simulink model "ConfiguredVirtualVehicleModel"  (R2023b)
settings: configuration reference "VehicleVariable" (kept outside this file)
StartFcn:
  | %tic
StopFcn:
  | %toc
model workspace (MAT data in the model file):
  ExtDrvCmdsSwitch : Simulink.Parameter (value not decoded)
  ExtDrvRefSwitch : Simulink.Parameter (value not decoded)
  ExtEnvSwitch : Simulink.Parameter (value not decoded)
  ExtGndSwitch : Simulink.Parameter (value not decoded)
values from neighbouring files (symbols this model uses):
  L = 2.79    [EVFmincon_custom.m]
symbols that are objects in the model workspace (value not decoded): ExtDrvCmdsSwitch, ExtDrvRefSwitch, ExtEnvSwitch, ExtGndSwitch
undefined symbols (not defined in the file or in its folder): AccelCmd, AmbTemp, BaroPress, CtrlTcuInitGear, CtrlVcuCltch1InitCmd, CurvGradRef, CurvRef, DCM, DecelCmd, Disabled, DriverAeroRes, DriverDrivelineRes, DriverInitialGear, DriverPreviewDist, DriverRollRes, DriverShiftTime, DriverTimeConst, DriverTractiveForce, EnvAbsPrs, EnvAirTemp, EnvGrvty, EnvNomFrictionScaling, EnvNominalGrade, EnvWindVelX, EnvWindVelY, EnvWindVelZ, FTP75, Gnd, Grade, HazzardCmd, HighBeamCmd, lambda_mux, LeftSignalCmd, LngRef, LowBeamCmd, LtrRef, PhiRef, PlntVehDstCGFrntAxl, PlntVehDstCGRearAxl, PlntVehInitLatPos, PlntVehInitLongPos, PlntVehInitPitchAng, PlntVehInitRollAng, PlntVehInitVertPos, PlntVehInitYawAng, PlntVehMass, PlntVehTrckWdth, PlntVehYawMomentInertia, PlntWhlLdRadius, RightSignalCmd, ScnCRMaxLatAccel, ScnCRRadius, ScnDLCGateLongPos, ScnDLCLatRef, ScnDLCLatRefOffset, ScnDLCLongRefBpt, ScnDLCLongRefStartPos, ScnDLCVehicleWidth, ScnFHCounterDwellTime, ScnFHInitialDwellTime ... (+22)
libraries: simulink x27, autolibutils x8, vehdynlibscenariocommon x7, vehdynlibviscommon x3, vehdynlibdriver x2, sim3dgroundtruthsensorlib x2, autolibshared x2, vrlib x1, autolibsharedcommon x1, sharedtransform x1, sim3dlib x1, sim3dautolib x1
(part 2 of 6)

== system ConfiguredVirtualVehicleModel/Controllers/Thermal Management ==
  CoolTemp : Inport
  CellTemps : Inport  Port=2
  No Control : Subsystem  VariantControl=No Control
  Thermal Control : ModelReference  ModelNameDialog=ThermalControl.slx  SimulationMode=Normal  VariantControl=Thermal Control  ModelReferenceVersion=1.43
  ValveCmd : Outport
  PumpCmd : Outport  Port=2

== system ConfiguredVirtualVehicleModel/Controllers/Thermal Output ==
  ValveCmd : Inport
  PumpCmd : Inport  Port=2
  Bus Creator : BusCreator  Inputs=2
  Thermal : Outport
  wires:
  PumpCmd/1 -> Bus Creator/2  "PumpCmd"
  ValveCmd/1 -> Bus Creator/1  "ValveCmd"
  Bus Creator/1 -> Thermal/1

== system ConfiguredVirtualVehicleModel/Controllers/Transmission Control Unit (TCU) ==
  Accel : Inport
  BrkCmd : Inport  Port=2
  GearReq : Inport  Port=3
  EngSpd : Inport  Port=4
  Omega : Inport  Port=5  Unit=rad/s
  VehSpdFdbk : Inport  Port=6
  ABSFlag : Inport  Port=7
  UpReq : Inport  Port=8
  DownReq : Inport  Port=9  Unit=rad/s
  DriverPassThrough : ModelReference  ModelNameDialog=DriverPassThrough  SimulationMode=Normal  VariantControl=DriverPassThrough  ModelReferenceVersion=7.0
  " Gear" : Outport  VectorParamsAs1DForOutWhenUnconnected=off

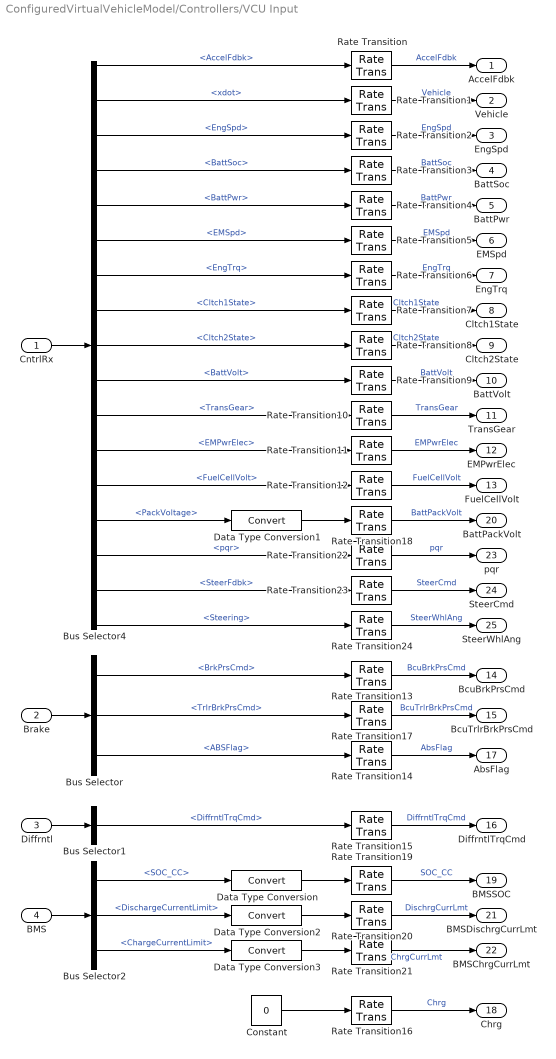
== system ConfiguredVirtualVehicleModel/Controllers/VCU Input ==
  CntrlRx : Inport
  Brake : Inport  Port=2
  Diffrntl : Inport  Port=3
  BMS : Inport  Port=4
  Bus Selector : BusSelector  OutputSignals=BrkPrsCmd,TrlrBrkPrsCmd,ABSFlag
  Bus Selector1 : BusSelector  OutputSignals=DiffrntlTrqCmd
  Bus Selector2 : BusSelector  OutputSignals=BMSInfo.SOC.SOC_CC,BMSCmd.CurrentLimitsBus.DischargeCurrentLimit,BMSCmd.CurrentLimitsBus.ChargeCurrentLimit
  Bus Selector4 : BusSelector  OutputSignals=Driver.AccelFdbk,Vehicle.xdot,Trans.EngSpd,Battery.BattSoc,Battery.BattPwr,Trans.EMSpd,Engine.EngTrq,Trans.Cltch1State,Trans.Cltch2State,Battery.BattVolt,Trans.TransGear,EM.EMPwrElec,FuelCell.FuelCellVolt,Battery.BMSSensors.PackVoltage,IMU.pqr,Driver.SteerFdbk,Steering
  Constant : Constant  Value=0  SampleTime=-1
  Data Type Conversion{,1..3} (4 alike) : DataTypeConversion  SaturateOnIntegerOverflow=off  RndMeth=Floor
  Rate Transition{,1..24} (25 alike) : RateTransition  Deterministic=off
  AccelFdbk : Outport
  Vehicle : Outport  Port=2
  EngSpd : Outport  Port=3
  BattSoc : Outport  Port=4
  BattPwr : Outport  Port=5
  EMSpd : Outport  Port=6
  EngTrq : Outport  Port=7
  Cltch1State : Outport  Port=8
  Cltch2State : Outport  Port=9
  BattVolt : Outport  Port=10
  TransGear : Outport  Port=11
  EMPwrElec : Outport  Port=12
  FuelCellVolt : Outport  Port=13
  BcuBrkPrsCmd : Outport  Port=14
  BcuTrlrBrkPrsCmd : Outport  Port=15
  DiffrntlTrqCmd : Outport  Port=16
  AbsFlag : Outport  Port=17
  Chrg : Outport  Port=18
  BMSSOC : Outport  Port=19
  BattPackVolt : Outport  Port=20
  BMSDischrgCurrLmt : Outport  Port=21
  BMSChrgCurrLmt : Outport  Port=22
  pqr : Outport  Port=23
  SteerCmd : Outport  Port=24
  SteerWhlAng : Outport  Port=25
  wires:
  Bus Selector4/5 -> Rate Transition4/1  "<BattPwr>"
  Bus Selector4/1 -> Rate Transition/1  "<AccelFdbk>"
  Bus Selector4/7 -> Rate Transition6/1  "<EngTrq>"
  Bus Selector4/4 -> Rate Transition3/1  "<BattSoc>"
  Bus Selector4/6 -> Rate Transition5/1  "<EMSpd>"
  CntrlRx/1 -> Bus Selector4/1
  Bus Selector4/11 -> Rate Transition10/1  "<TransGear>"
  Bus Selector4/9 -> Rate Transition8/1  "<Cltch2State>"
  Bus Selector4/13 -> Rate Transition12/1  "<FuelCellVolt>"
  Bus Selector4/2 -> Rate Transition1/1  "<xdot>"
  Bus Selector4/8 -> Rate Transition7/1  "<Cltch1State>"
  Bus Selector4/10 -> Rate Transition9/1  "<BattVolt>"
  Bus Selector4/3 -> Rate Transition2/1  "<EngSpd>"
  Bus Selector4/12 -> Rate Transition11/1  "<EMPwrElec>"
  Bus Selector/1 -> Rate Transition13/1  "<BrkPrsCmd>"
  Constant/1 -> Rate Transition16/1
  Brake/1 -> Bus Selector/1
  Bus Selector/3 -> Rate Transition14/1  "<ABSFlag>"
  Diffrntl/1 -> Bus Selector1/1
  Bus Selector1/1 -> Rate Transition15/1  "<DiffrntlTrqCmd>"
  Rate Transition/1 -> AccelFdbk/1  "AccelFdbk"
  Rate Transition1/1 -> Vehicle/1  "Vehicle"
  Rate Transition2/1 -> EngSpd/1  "EngSpd"
  Rate Transition3/1 -> BattSoc/1  "BattSoc"
  Rate Transition4/1 -> BattPwr/1  "BattPwr"
  Rate Transition5/1 -> EMSpd/1  "EMSpd"
  Rate Transition6/1 -> EngTrq/1  "EngTrq"
  Rate Transition7/1 -> Cltch1State/1  "Cltch1State"
  Rate Transition8/1 -> Cltch2State/1  "Cltch2State"
  Rate Transition9/1 -> BattVolt/1  "BattVolt"
  Rate Transition10/1 -> TransGear/1  "TransGear"
  Rate Transition11/1 -> EMPwrElec/1  "EMPwrElec"
  Rate Transition12/1 -> FuelCellVolt/1  "FuelCellVolt"
  Rate Transition13/1 -> BcuBrkPrsCmd/1  "BcuBrkPrsCmd"
  Rate Transition14/1 -> AbsFlag/1  "AbsFlag"
  Rate Transition15/1 -> DiffrntlTrqCmd/1  "DiffrntlTrqCmd"
  Rate Transition16/1 -> Chrg/1  "Chrg"
  Rate Transition20/1 -> BMSDischrgCurrLmt/1  "DischrgCurrLmt"
  Rate Transition19/1 -> BMSSOC/1  "SOC_CC"
  Rate Transition21/1 -> BMSChrgCurrLmt/1  "ChrgCurrLmt"
  Data Type Conversion3/1 -> Rate Transition21/1
  Data Type Conversion2/1 -> Rate Transition20/1
  Bus Selector2/1 -> Data Type Conversion/1  "<SOC_CC>"
  Data Type Conversion/1 -> Rate Transition19/1
  Bus Selector2/3 -> Data Type Conversion3/1  "<ChargeCurrentLimit>"
  Bus Selector2/2 -> Data Type Conversion2/1  "<DischargeCurrentLimit>"
  BMS/1 -> Bus Selector2/1
  Data Type Conversion1/1 -> Rate Transition18/1
  Rate Transition18/1 -> BattPackVolt/1  "BattPackVolt"
  Bus Selector4/14 -> Data Type Conversion1/1  "<PackVoltage>"
  Bus Selector/2 -> Rate Transition17/1  "<TrlrBrkPrsCmd>"
  Rate Transition17/1 -> BcuTrlrBrkPrsCmd/1  "BcuTrlrBrkPrsCmd"
  Rate Transition22/1 -> pqr/1  "pqr"
  Rate Transition23/1 -> SteerCmd/1  "SteerCmd"
  Rate Transition24/1 -> SteerWhlAng/1  "SteerWhlAng"
  Bus Selector4/15 -> Rate Transition22/1  "<pqr>"
  Bus Selector4/16 -> Rate Transition23/1  "<SteerFdbk>"
  Bus Selector4/17 -> Rate Transition24/1  "<Steering>"

== system ConfiguredVirtualVehicleModel/Controllers/VCU Output ==
  EngTrqCmd : Inport
  EMTrqCmd : Inport  Port=2
  VcuBrkPrsCmd : Inport  Port=3
  VcuTrlrBrkPrsCmd : Inport  Port=4
  Cltch1Cmd : Inport  Port=5
  Neutral : Inport  Port=6
  FuelCellCurrCmd : Inport  Port=7
  FuelCellTempCmd : Inport  Port=8
  Bus Creator5 : BusCreator  Inputs=8
  Vcu : Outport
  wires:
  Cltch1Cmd/1 -> Bus Creator5/5  "Cltch1Cmd"
  EngTrqCmd/1 -> Bus Creator5/1  "EngTrqCmd"
  Bus Creator5/1 -> Vcu/1  "Vcu"
  VcuBrkPrsCmd/1 -> Bus Creator5/3  "VcuBrkPrsCmd"
  Neutral/1 -> Bus Creator5/6  "Neutral"
  FuelCellCurrCmd/1 -> Bus Creator5/7  "FuelCellCurrCmd"
  EMTrqCmd/1 -> Bus Creator5/2  "EMTrqCmd"
  FuelCellTempCmd/1 -> Bus Creator5/8  "FuelCellTempCmd"
  VcuTrlrBrkPrsCmd/1 -> Bus Creator5/4  "VcuTrlrBrkPrsCmd"

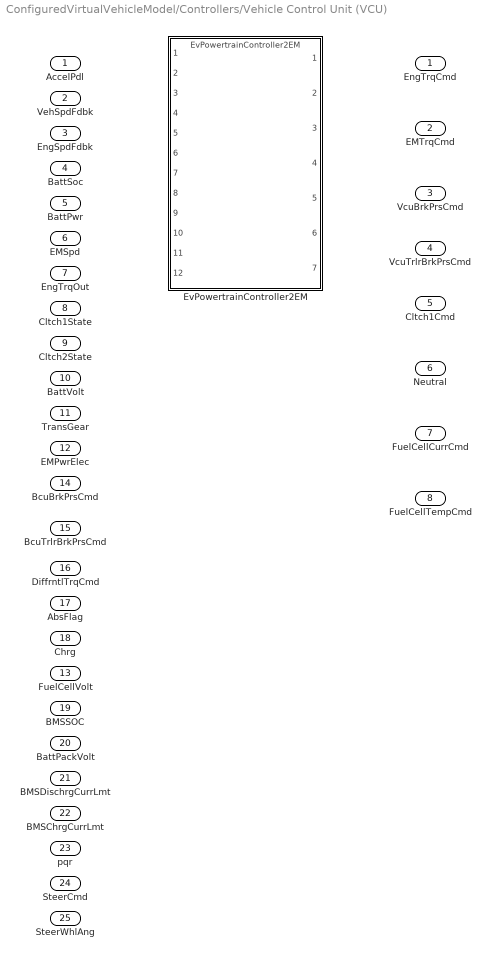
== system ConfiguredVirtualVehicleModel/Controllers/Vehicle Control Unit (VCU) ==
  AccelPdl : Inport
  VehSpdFdbk : Inport  Port=2
  EngSpdFdbk : Inport  Port=3
  BattSoc : Inport  Port=4
  BattPwr : Inport  Port=5
  EMSpd : Inport  Port=6
  EngTrqOut : Inport  Port=7
  Cltch1State : Inport  Port=8
  Cltch2State : Inport  Port=9
  BattVolt : Inport  Port=10
  TransGear : Inport  Port=11
  EMPwrElec : Inport  Port=12
  FuelCellVolt : Inport  Port=13
  BcuBrkPrsCmd : Inport  Port=14
  BcuTrlrBrkPrsCmd : Inport  Port=15
  DiffrntlTrqCmd : Inport  Port=16
  AbsFlag : Inport  Port=17
  Chrg : Inport  Port=18
  BMSSOC : Inport  Port=19
  BattPackVolt : Inport  Port=20
  BMSDischrgCurrLmt : Inport  Port=21
  BMSChrgCurrLmt : Inport  Port=22
  pqr : Inport  Port=23
  SteerCmd : Inport  Port=24
  SteerWhlAng : Inport  Port=25
  EvPowertrainController2EM : ModelReference  ModelNameDialog=EvPowertrainController2EM  SimulationMode=Normal  VariantControl=EvPowertrainController2EM  ModelReferenceVersion=7.70
  EngTrqCmd : Outport  VectorParamsAs1DForOutWhenUnconnected=off
  EMTrqCmd : Outport  Port=2  VectorParamsAs1DForOutWhenUnconnected=off
  VcuBrkPrsCmd : Outport  Port=3  VectorParamsAs1DForOutWhenUnconnected=off
  VcuTrlrBrkPrsCmd : Outport  Port=4  VectorParamsAs1DForOutWhenUnconnected=off
  Cltch1Cmd : Outport  Port=5  VectorParamsAs1DForOutWhenUnconnected=off
  Neutral : Outport  Port=6  VectorParamsAs1DForOutWhenUnconnected=off
  FuelCellCurrCmd : Outport  Port=7  VectorParamsAs1DForOutWhenUnconnected=off
  FuelCellTempCmd : Outport  Port=8  VectorParamsAs1DForOutWhenUnconnected=off

== system ConfiguredVirtualVehicleModel/Driver Commands/Driver Commands ==
  VehRef : Inport
  VehFdbk : Inport  Port=2
  Env : Inport  Port=3
  SteerCmd : Inport  Port=4
  AccelCmd : Inport  Port=5
  BrakeCmd : Inport  Port=6
  GearCmd : Inport  Port=7
  Dashboard Widgets : Subsystem  VariantControl=driverType==5
  Game Wheel Hardware : Subsystem  VariantControl=driverType==6
  Longitudinal Driver : Subsystem  VariantControl=driverType==1
  No Driver : Subsystem  VariantControl=driverType==7
  Open Loop : Subsystem  VariantControl=driverType==4
  Predictive Driver : Subsystem  VariantControl=driverType==2
  Predictive Stanley Driver : Subsystem  VariantControl=driverType==3
  " Driver" : Outport  VectorParamsAs1DForOutWhenUnconnected=off

== system ConfiguredVirtualVehicleModel/Environment/Ground Feedback ==
  Friction : Inport
  WheelFdbk : Inport  Port=2
  3D Engine : Subsystem  VariantControl=1
  Constant : Subsystem  VariantControl=0
  Three-Axle Constant : Subsystem  VariantControl=2
  Gnd : Outport  VectorParamsAs1DForOutWhenUnconnected=off

== system ConfiguredVirtualVehicleModel/Environment/Subsystem ==
  ExtEnv : Inport
  ExtGnd : Inport  Port=2
  AmbTemp : Inport  Port=3
  BaroPress : Inport  Port=4
  Wind : Inport  Port=5
  InGnd : Inport  Port=6
  Bus Assignment : BusAssignment  AssignedSignals=AmbTemp,BaroPress,Wind,Grade
  Bus Assignment1 : BusAssignment  AssignedSignals=Z,DCM,lambda_mux
  Bus Assignment2 : BusAssignment  AssignedSignals=BaroPress,AmbTemp,Wind,Grade,Gnd
  Bus Selector : BusSelector  OutputSignals=BaroPress,AmbTemp,Wind,Grade
  Estimated Grade : Subsystem
  ExtEnvSwitch : Constant  Value=ExtEnvSwitch  SampleTime=-1
  ExtGndSwitch : Constant  Value=ExtGndSwitch  SampleTime=-1
  Switch : Switch  Criteria=u2 > Threshold  SaturateOnIntegerOverflow=off  InputSameDT=off
  Switch1 : Switch  Criteria=u2 > Threshold  SaturateOnIntegerOverflow=off  InputSameDT=off
  To Virtual Bus : SignalConversion  ConversionOutput=Virtual bus  OverrideOpt=off
  VVCEnv : Constant  Value=0  OutDataTypeStr=Bus: VVCEnvGnd  SampleTime=-1
  Variant Subsystem : Subsystem  Variant=on  VariantControlMode=label  LabelModeActiveChoice=TwoAxle
  Env : Outport
  wires:
  Bus Assignment1/1 -> Switch1/3
  Estimated Grade/1(Grade) -> Bus Assignment/5
  ExtGndSwitch/1 -> Switch1/2
  ExtEnv/1 -> Switch/1, Bus Assignment/1
  InGnd/1 -> Variant Subsystem/1(InGnd), Estimated Grade/1(Gnd)
  ExtEnvSwitch/1 -> Switch/2
  Bus Assignment/1 -> Switch/3
  BaroPress/1 -> Bus Assignment/3
  VVCEnv/1 -> Bus Assignment2/1
  Switch1/1 -> Bus Assignment2/6
  ExtGnd/1 -> Switch1/1, Bus Assignment1/1
  Wind/1 -> Bus Assignment/4
  Bus Selector/1 -> Bus Assignment2/2  "<BaroPress>"
  Switch/1 -> Bus Selector/1
  Bus Selector/2 -> Bus Assignment2/3  "<AmbTemp>"
  Bus Assignment2/1 -> To Virtual Bus/1
  Bus Selector/4 -> Bus Assignment2/5  "<Grade>"
  Bus Selector/3 -> Bus Assignment2/4  "<Wind>"
  AmbTemp/1 -> Bus Assignment/2
  To Virtual Bus/1 -> Env/1
  Variant Subsystem/1(z) -> Bus Assignment1/2
  Variant Subsystem/2(<DCM>) -> Bus Assignment1/3
  Variant Subsystem/3(lambda_mux) -> Bus Assignment1/4

== system ConfiguredVirtualVehicleModel/Environment/Varying Friction ==
  In1 : Inport
  In2 : Inport  Port=2
  Cg : Inport  Port=3
  Constant Friction : Subsystem  VariantControl=0
  Three-Axle Constant Friction : Subsystem  VariantControl=2
  Varying Friction : Subsystem  VariantControl=1
  FricCoeffLambda : Outport

== system ConfiguredVirtualVehicleModel/Scenarios/Coordinate Systems ==
  ExtDrvRefIn : Inport
  ExtDrvCmdIn : Inport  Port=2
  ISO 8855 (Z-up) : Subsystem  VariantControl=Choice
  SAE J670 (Z-down) : Subsystem  VariantControl=ISO 8855 (Z-up)1
  ExtDrvRef : Outport
  ExtDrvCmd : Outport  Port=2

== system ConfiguredVirtualVehicleModel/Scenarios/Reference Generator ==
  note: 1) Add Subsystem or Model blocks as valid variant choices.
      | 2) You cannot connect blocks at this level. At simulation, connectivity is automatically
      | determined, based on the active variant and port name matching.
  VehFdbk : Inport
  Reference Generator : Subsystem  Priority=1  VariantControl=Vehicle Dynamic Scenarios  mask(Reference Generator){manType=Drive Cycle, manOverride=off, prevType=Drive Cycle, t_start=ScnStartTime, xdot_r=ScnLongVelRef, xdotUnit=mph, steerDir=off, aMode=2, omega_hw=ScnISHandwheelRate, theta_max=ScnISMaxHandwheelAng, t_stop=ScnISSteerHoldTime, ay_max=ScnISMaxLatAccel, ay_stop=on, XGate=ScnDLCGateLongPos, xStart=ScnDLCLongRefStartPos, vehW=ScnDLCVehicleWidth, latoff=ScnDLCLatRefOffset, latRefbp=ScnDLCLongRefBpt, latRef=ScnDLCLatRef, t_sweep=ScnSSSweepTime, theta_hw=ScnSSSteerAmp, theta_hw_final=ScnSSFinalFreq, steerF=ScnSDSteerFreq, steerA=ScnSDSteerAmp, tdwell=ScnSDDwellTime, R=ScnCRRadius, cr_ay_max=ScnCRMaxLatAccel, cr_ay_stop=off, steerRate=ScnFHSteerSpeed, steerAFH=ScnFHSteerAmp, pFdbk=off, tDwell1=ScnFHInitialDwellTime, tDwell2=ScnFHCounterDwellTime, tSteer3=ScnFHReturnTime, pZero=ScnFHRollRateZeroCross, cycleVar=FTP75, ax=.5, ax_dec=.5, fixhw=on, x_brake=175, t_wot2=20, simTime=ScnSimTime, engine3D=Disabled, SceneDesc=Open surface, dt3D=.03, defaultPos=User-specified, X_o=PlntVehInitLongPos, Y_o=PlntVehInitLatPos, Z_o=PlntVehInitVertPos, phi_o=PlntVehInitRollAng, theta_o=PlntVehInitPitchAng, psi_o=PlntVehInitYawAng}
      mask prompts: manType "vdynblks:vehdynManConstantRadius:blkPrm_manType"; manOverride "vdynblks:vehdynManConstantRadius:blkPrm_manOverride"; t_start "vdynblks:vehdynManConstantRadius:blkPrm_t_start"; xdot_r "vdynblks:vehdynManConstantRadius:blkPrm_xdot_r"; xdotUnit "vdynblks:vehdynManStraightBrake:blkPrm_xdotUnit"; steerDir "Change direction, steerDir"; omega_hw "vdynblks:vehdynManConstantRadius:blkPrm_omega_hw"; theta_max "vdynblks:vehdynManConstantRadius:blkPrm_theta_max"; t_stop "vdynblks:vehdynManConstantRadius:blkPrm_t_stop"; ay_max "vdynblks:vehdynManConstantRadius:blkPrm_ay_max"; ay_stop "vdynblks:vehdynManConstantRadius:blkPrm_ay_stop"; XGate "vdynblks:vehdynManConstantRadius:blkPrm_XGate"; xStart "vdynblks:vehdynManConstantRadius:blkPrm_xStart"; vehW "vdynblks:vehdynManConstantRadius:blkPrm_vehW"; latoff "vdynblks:vehdynManConstantRadius:blkPrm_latoff"; latRefbp "vdynblks:vehdynManConstantRadius:blkPrm_latRefbp"; latRef "vdynblks:vehdynManConstantRadius:blkPrm_latRef"; t_sweep "vdynblks:vehdynManConstantRadius:blkPrm_t_sweep"; theta_hw "vdynblks:vehdynManConstantRadius:blkPrm_theta_hw"; theta_hw_final "vdynblks:vehdynManConstantRadius:blkPrm_theta_hw_final"; steerF "vdynblks:vehdynManConstantRadius:blkPrm_steerF"; steerA "vdynblks:vehdynManConstantRadius:blkPrm_steerA"; tdwell "vdynblks:vehdynManConstantRadius:blkPrm_tdwell"; R "Radius value, R [m]:"; cr_ay_max "Lateral acceleration absolute threshold, ay_max [g]:"; cr_ay_stop "Stop simulation at lateral acceleration threshold"; steerRate "vdynblks:vehdynManFishook:blkPrm_steerRate"; steerAFH "vdynblks:vehdynManConstantRadius:blkPrm_steerAFH"; pFdbk "vdynblks:vehdynManFishook:blkPrm_pFdbk"; tDwell1 "vdynblks:vehdynManFishook:blkPrm_tDwell1"; tDwell2 "vdynblks:vehdynManFishook:blkPrm_tDwell2"; tSteer3 "vdynblks:vehdynManFishook:blkPrm_tSteer3"; pZero "vdynblks:vehdynManFishook:blkPrm_pZero"; cycleVar "autoblks_shared:autoblkDriveCycleSource:blkPrm_cycleVar"; ax "vdynblks:vehdynManStraightBrake:blkPrm_ax"; ax_dec "vdynblks:vehdynManStraightBrake:blkPrm_ax_dec"; fixhw "vdynblks:vehdynManStraightBrake:blkPrm_fixhw"; x_brake "vdynblks:vehdynManStraightBrake:blkPrm_x_brake"; t_wot2 "autoblks_shared:autoblkDriveCycleSource:blkPrm_t_wot2"; simTime "vdynblks:vehdynManConstantRadius:blkPrm_simTime"; engine3D "vdynblks:vehdynManConstantRadius:blkPrm_engine3D"; SceneDesc "vdynblks:vehdynManConstantRadius:blkPrm_SceneDesc"; dt3D "vdynblks:vehdynManConstantRadius:blkPrm_dt3D"; X_o "Initial longitudinal position, X_o [m]:"; Y_o "Initial lateral position, Y_o [m]:"; Z_o "vdynblks:vehdynManConstantRadius:blkPrm_Z_o"; phi_o "vdynblks:vehdynManConstantRadius:blkPrm_phi_o"; theta_o "vdynblks:vehdynManConstantRadius:blkPrm_theta_o"; psi_o "Initial yaw angle, psi_o [rad]:"
      mask help: vdynblks:vehdynManConstantRadius:blkDesc
      mask init:
      | [~]=vdynblksrefconfig(gcb,0);
      settings: AttributesFormatString=%<manType>
      mask Help: eval('vdynblkshelp(''vdcrrefgen'')');
      mask TypeOptions manType: autoblks_reference:autoVirtualRefGen:blkCmb_manType_c1 | autoblks_reference:autoVirtualRefGen:blkCmb_manType_c2 | autoblks_reference:autoVirtualRefGen:blkCmb_manType_c3 | autoblks_reference:autoVirtualRefGen:blkCmb_manType_c4 | autoblks_reference:autoVirtualRefGen:blkCmb_manType_c5 | autoblks_reference:autoVirtualRefGen:blkCmb_manType_c6 | autoblks_reference:autoVirtualRefGen:blkCmb_manType_c7 | autoblks_reference:autoVirtualRefGen:blkCmb_manType_c8 | autoblks_reference:autoVirtualRefGen:blkCmb_manType_c9 | autoblks_reference:autoVirtualRefGen:blkCmb_manType_c10
      mask Callback manType:
      | [~]=vdynblksrefconfig(gcb,0);
      | [~]=vdynblksrefconfig(gcb,1);
      mask Callback manOverride: [~]=vdynblksrefconfig(gcb,3);
      mask TypeOptions prevType: autoblks_reference:autoVirtualRefGen:blkCmb_manType_c1 | autoblks_reference:autoVirtualRefGen:blkCmb_manType_c2 | autoblks_reference:autoVirtualRefGen:blkCmb_manType_c3 | autoblks_reference:autoVirtualRefGen:blkCmb_manType_c4 | autoblks_reference:autoVirtualRefGen:blkCmb_manType_c5 | autoblks_reference:autoVirtualRefGen:blkCmb_manType_c6 | autoblks_reference:autoVirtualRefGen:blkCmb_manType_c7 | autoblks_reference:autoVirtualRefGen:blkCmb_manType_c8 | autoblks_reference:autoVirtualRefGen:blkCmb_manType_c9 | autoblks_reference:autoVirtualRefGen:blkCmb_manType_c10
      mask TypeOptions xdotUnit:
      | Reference Generator/Braking/Straight Maneuver Reference
      | Generator/xdotUnit | Reference Generator/Constant Radius/Constant Radius/xdotUnit | Reference Generator/Double Lane Change/Double Lane Change/xdotUnit | Reference Generator/Fishhook/Fishhook/xdotUnit | Reference Generator/Increasing Steer/Increasing Steer/xdotUnit | Reference Generator/Sine with Dwell/Sine With Dwell/xdotUnit | Reference Generator/Swept Sine/Swept Sine/xdotUnit | Reference Generator/WOT/Drive Cycle Source/srcUnit
      mask TypeOptions steerDir: Reference Generator/Constant Radius/Constant Radius/steerDir | Reference Generator/Fishhook/Fishhook/steerDir | Reference Generator/Increasing Steer/Increasing Steer/steerDir | Reference Generator/Sine with Dwell/Sine With Dwell/steerDir
      mask TypeOptions omega_hw: Reference Generator/Increasing Steer/Increasing Steer/omega_hw
      mask TypeOptions theta_max: Reference Generator/Increasing Steer/Increasing Steer/theta_max
      mask TypeOptions t_stop: Reference Generator/Increasing Steer/Increasing Steer/t_stop
      mask TypeOptions ay_max: Reference Generator/Increasing Steer/Increasing Steer/ay_max
      mask TypeOptions ay_stop: Reference Generator/Increasing Steer/Increasing Steer/ay_stop
      mask Callback ay_stop:
      | if strcmp(get_param(gcb,'ay_stop'),'off')
      |     autoblksenableparameters(gcb, [], {'ay_max'},[],[],true);
      | else
      |     autoblksenableparameters(gcb,{'ay_max'},[],[],[],true);
      | end
      mask TypeOptions XGate: Reference Generator/Double Lane Change/Double Lane Change/XGate
      mask TypeOptions xStart: Reference Generator/Double Lane Change/Double Lane Change/xStart
      mask TypeOptions vehW: Reference Generator/Double Lane Change/Double Lane Change/vehW
      mask TypeOptions latoff: Reference Generator/Double Lane Change/Double Lane Change/latoff
      mask TypeOptions latRefbp: Reference Generator/Double Lane Change/Double Lane Change/latRefbp
      mask TypeOptions latRef: Reference Generator/Double Lane Change/Double Lane Change/latRef
      mask TypeOptions t_sweep: Reference Generator/Swept Sine/Swept Sine/t_sweep
      mask TypeOptions theta_hw: Reference Generator/Swept Sine/Swept Sine/theta_hw
      mask TypeOptions theta_hw_final: Reference Generator/Swept Sine/Swept Sine/theta_hw_final
      mask TypeOptions steerF: Reference Generator/Sine with Dwell/Sine With Dwell/steerF
      mask TypeOptions steerA: Reference Generator/Sine with Dwell/Sine With Dwell/steerA
      mask TypeOptions tdwell: Reference Generator/Sine with Dwell/Sine With Dwell/tdwell
      mask TypeOptions R: Reference Generator/Constant Radius/Constant Radius/R
      mask TypeOptions cr_ay_max: Reference Generator/Constant Radius/Constant Radius/ay_max
      mask TypeOptions cr_ay_stop: Reference Generator/Constant Radius/Constant Radius/ay_stop
      mask TypeOptions steerRate: Reference Generator/Fishhook/Fishhook/steerRate
      mask TypeOptions pFdbk: Reference Generator/Fishhook/Fishhook/pFdbk
      mask Callback pFdbk:
      | block = gcb;
      | pFdbkChk = get_param(block,'pFdbk');
      | if strcmp(pFdbkChk,'off')
      |     autoblksenableparameters(block,{'tDwell1'},{'pZero'},[],[],'false')
      | else
      |     autoblksenableparameters(block,{'pZero'},{'tDwell1'},[],[],'false')
      | end
      mask TypeOptions tDwell1: Reference Generator/Fishhook/Fishhook/tDwell1
      mask TypeOptions tDwell2: Reference Generator/Fishhook/Fishhook/tDwell2
      mask TypeOptions tSteer3: Reference Generator/Fishhook/Fishhook/tSteer3
      mask TypeOptions pZero: Reference Generator/Fishhook/Fishhook/pZero
      mask TypeOptions cycleVar: Reference Generator/Drive Cycle/Drive Cycle Source/cycleVar
      mask TypeOptions ax:
      | Reference Generator/Braking/Straight Maneuver Reference
      | Generator/ax
      mask TypeOptions ax_dec:
      | Reference Generator/Braking/Straight Maneuver Reference
      | Generator/ax_dec
      mask TypeOptions fixhw:
      | Reference Generator/Braking/Straight Maneuver Reference
      | Generator/fixhw
      mask TypeOptions x_brake:
      | Reference Generator/Braking/Straight Maneuver Reference
      | Generator/x_brake
      mask TypeOptions t_wot2: Reference Generator/WOT/Drive Cycle Source/t_wot2
      mask TypeOptions engine3D: 3D Engine/engine3D
      mask Callback engine3D: [~]=vdynblksrefconfig(gcb,4);
      mask TypeOptions SceneDesc: 3D Engine/SceneDesc
      mask Callback SceneDesc: [~] = vdynblks3Dsceneconfig(gcb);
      mask TypeOptions dt3D: 3D Engine/dt3D
      mask TypeOptions defaultPos: Recommended for scene | User-specified
      mask Callback defaultPos: [~] = vdynblksmdlWSconfig(gcb,false);
      mask TypeOptions X_o: 3D Engine/X_o | Reference Generator/Constant Radius/Constant Radius/X_o | Reference Generator/Double Lane Change/Double Lane Change/X_o | Reference Generator/Increasing Steer/Increasing Steer/X_o | Reference Generator/Sine with Dwell/Sine With Dwell/X_o | Reference Generator/Swept Sine/Swept Sine/X_o
      mask TypeOptions Y_o: 3D Engine/Y_o | Reference Generator/Constant Radius/Constant Radius/Y_o | Reference Generator/Double Lane Change/Double Lane Change/Y_o | Reference Generator/Fishhook/Fishhook/Y_o | Reference Generator/Increasing Steer/Increasing Steer/Y_o | Reference Generator/Sine with Dwell/Sine With Dwell/Y_o | Reference Generator/Swept Sine/Swept Sine/Y_o
      mask TypeOptions Z_o: 3D Engine/Z_o
      mask TypeOptions phi_o: 3D Engine/phi_o | Reference Generator/Double Lane Change/Double Lane Change/psi_o
      mask TypeOptions theta_o: 3D Engine/theta_o
      mask TypeOptions psi_o: 3D Engine/psi_o | Reference Generator/Constant Radius/Constant Radius/psi_o | Reference Generator/Fishhook/Fishhook/psi_o | Reference Generator/Increasing Steer/Increasing Steer/psi_o | Reference Generator/Sine with Dwell/Sine With Dwell/psi_o | Reference Generator/Swept Sine/Swept Sine/psi_o
      mask DialogControl modTab Prompt: vdynblks:vehdynManConstantRadius:blkDlg_modTab
      mask DialogControl configGroup Prompt: vdynblks:vehdynManConstantRadius:blkDlg_configGroup
      mask DialogControl manType Prompt: Maneuver:
      mask DialogControl manOverride Prompt: Use maneuver-specific driver, initial position, and scene
      mask DialogControl t_start Prompt: Maneuver start time, t_start [s]:
      mask DialogControl xdot_r Prompt: Longitudinal velocity reference, xdot_r:
      mask DialogControl xdotUnit Prompt: Units of velocity, xdotUnit []:
      mask DialogControl ISGroup Prompt: vdynblks:vehdynManConstantRadius:blkDlg_ISGroup
      mask DialogControl omega_hw Prompt: Handwheel rate, omega_hw [deg/s]:
      mask DialogControl theta_max Prompt: Maximum handwheel angle, theta_max [deg]:
      mask DialogControl t_stop Prompt: Steering hold time after max angle reached, t_stop [s]:
      mask DialogControl ay_max Prompt: Lateral acceleration threshold, ay_max [g]:
      mask DialogControl ay_stop Prompt: Stop simulation at lateral acceleration threshold:
      mask DialogControl DLCGroup Prompt: vdynblks:vehdynManConstantRadius:blkDlg_DLCGroup
      mask DialogControl XGate Prompt: Inertial longitudinal position of gate entrance, XGate [m]:
      mask DialogControl xStart Prompt: Distance after target speed to begin reference, xStart [m]:
      mask DialogControl vehW Prompt: Vehicle width, vehW [m]:
      mask DialogControl latoff Prompt: Lateral offset, latoff [m]:
      mask DialogControl latRefbp Prompt: Lateral reference position breakpoints [m]:
      mask DialogControl latRef Prompt: Lateral reference data, latRef [m]:
      mask DialogControl SSGroup Prompt: vdynblks:vehdynManConstantRadius:blkDlg_SSGroup
      mask DialogControl t_sweep Prompt: Swept time, t_sweep [s]:
      mask DialogControl theta_hw Prompt: Steering amplitude, theta_hw [deg]:
      mask DialogControl theta_hw_final Prompt: Final frequency, theta_hw_final [Hz]:
      mask DialogControl SDGroup Prompt: vdynblks:vehdynManConstantRadius:blkDlg_SDGroup
      mask DialogControl steerF Prompt: Steer frequency, steerF [Hz]:
      mask DialogControl steerA Prompt: Steer amplitude, steerA [deg]:
      mask DialogControl tdwell Prompt: Dwell time, tdwell [s]:
      mask DialogControl CRGroup Prompt: vdynblks:vehdynManConstantRadius:blkDlg_CRGroup
      mask DialogControl FHGroup Prompt: vdynblks:vehdynManConstantRadius:blkDlg_FHGroup
      mask DialogControl steerRate Prompt: Steer and countersteer speed, steerRate [deg/s]:
      mask DialogControl steerAFH Prompt: Steer amplitude, steerAFH, [deg]:
      mask DialogControl pFdbk Prompt: Use roll rate to determine initial steer dwell time
      mask DialogControl tDwell1 Prompt: Initial dwell time, tDwell1 [s]:
      mask DialogControl tDwell2 Prompt: Countersteer dwell time, tDwell2 [s]:
      mask DialogControl tSteer3 Prompt: Return to center time, tSteer3 [s]:
      mask DialogControl pZero Prompt: Roll rate countersteer initiation zero crossing threshold, pZero [deg/s]:
      mask DialogControl pZero Tooltip: vdynblks:vehdynManFishook:blkDlg_pZeroToolTip
      mask DialogControl DCGroup Prompt: Drive Cycle
      mask DialogControl cycleVar Prompt: Drive cycle source:
      mask DialogControl openDCbutton Prompt: Click for all configuration options
      mask DialogControl openDCbutton Callback: open_system([gcb '/Reference Generator/Drive Cycle/Drive Cycle Source'])
      mask DialogControl BGroup Prompt: Braking
      mask DialogControl ax Prompt: Longitudinal acceleration at t_start, ax [g]:
      mask DialogControl ax_dec Prompt: Longitudinal deceleration at t_brake, ax_dec [g]:
      mask DialogControl fixhw Prompt: Set handwheel angle to 0 deg after braking
      mask DialogControl x_brake Prompt: Longitudinal displacement of vehicle CG, x_brake [m]:
      mask DialogControl WOTGroup Prompt: Wide Open Throttle (WOT)
      mask DialogControl t_wot2 Prompt: Time to start deceleration, t_wot2 [s]:
      mask DialogControl simTime Prompt: Simulation time, simTime [s]:
      mask DialogControl simUpdate Prompt: vdynblks:vehdynManConstantRadius:blkDlg_simUpdate
      mask DialogControl simUpdate Callback: [~]=vdynblksrefconfig(gcb,2);
      mask DialogControl sim3DTab Prompt: vdynblks:vehdynManConstantRadius:blkDlg_sim3DTab
      mask DialogControl sim3DGroup Prompt: vdynblks:vehdynManConstantRadius:blkDlg_sim3DGroup
      mask DialogControl engine3D Prompt: 3D Engine:
      mask DialogControl SceneDesc Prompt: Scene:
      mask DialogControl dt3D Prompt: 3D Engine frame rate, dt3D [s]:
      mask DialogControl posSetupDesc Prompt: To use these initial vehicle positions, first Apply the initial values and then click Update the model workspaces with the initial values.
      mask DialogControl Z_o Prompt: Initial vertical position, Z_o [m]:
      mask DialogControl phi_o Prompt: Initial roll angle, phi_o [rad]:
      mask DialogControl theta_o Prompt: Initial pitch angle, theta_o [rad]:
      mask Display: image('vdbslibscen.png')
  Ref : Outport
  Vis : Outport  Port=2
  Fdbk : Outport  Port=3

== system ConfiguredVirtualVehicleModel/Scenarios/Reference Routing ==
  ExtDrvRef : Inport  OutDataTypeStr=Bus: VVCDrvRef
  ExtDrvCmds : Inport  Port=2  OutDataTypeStr=Bus: VVCDrvCmd
  ScenBus : Inport  Port=3
  Bus Assignment : BusAssignment  AssignedSignals=LngRef,LtrRef,XRef,YRef,PhiRef,CurvRef
  Bus Assignment1 : BusAssignment  AssignedSignals=SteerCmd.EnblSteerCmd,SteerCmd.SteerCmd,SteerCmd.SteerHld,SteerCmd.SteerZero,AccelCmd.EnblAccelCmd,AccelCmd.AccelCmd,AccelCmd.AccelHld,AccelCmd.AccelZero,DecelCmd.EnblDecelCmd,DecelCmd.DecelCmd,DecelCmd.DecelHld,DecelCmd.DecelZero
  Bus Creator : BusCreator  Inputs=2
  Bus Selector : BusSelector  OutputSignals=LngRef,LtrlRef,PoseRef,CurvRef
  Bus Selector1 : BusSelector  OutputSignals=EnblSteerCmd,SteerOvrCmd,SteerHld,SteerZero,EnblAccelOvr,AccelOvrCmd,AccelHld,AccelZero,EnblDecelCmd,DecelOvrCmd,DecelHld,DecelZero
  Demux : Demux  Outputs=3
  ExtDrvCmdsSwitch : Constant  Value=ExtDrvCmdsSwitch
  ExtDrvRefSwitch : Constant  Value=ExtDrvRefSwitch
  Switch : Switch  Criteria=u2 > Threshold  SaturateOnIntegerOverflow=off  InputSameDT=off
  Switch1 : Switch  Criteria=u2 > Threshold  SaturateOnIntegerOverflow=off  InputSameDT=off
  Unit Conversion1 : UnitConversion
  Unit Conversion2 : UnitConversion
  VehRef : Outport
  wires:
  Bus Selector1/9 -> Bus Assignment1/10  "<EnblDecelCmd>"
  Bus Selector/3 -> Demux/1  "<PoseRef>"
  Bus Selector/1 -> Unit Conversion2/1  "<LngRef>"
  Bus Selector1/8 -> Bus Assignment1/9  "<AccelZero>"
  Demux/2 -> Bus Assignment/5
  Bus Selector1/4 -> Bus Assignment1/5  "<SteerZero>"
  Bus Selector1/3 -> Bus Assignment1/4  "<SteerHld>"
  Bus Selector1/10 -> Bus Assignment1/11  "<DecelOvrCmd>"
  ExtDrvRef/1 -> Bus Assignment/1, Switch/1
  Bus Selector1/1 -> Bus Assignment1/2  "<EnblSteerCmd>"
  Bus Assignment/1 -> Switch/3
  Demux/1 -> Bus Assignment/4
  Demux/3 -> Bus Assignment/6
  Bus Assignment1/1 -> Switch1/3
  Bus Selector/2 -> Bus Assignment/3  "<LtrlRef>"
  Bus Selector1/7 -> Bus Assignment1/8  "<AccelHld>"
  ScenBus/1 -> Bus Selector1/1, Bus Selector/1
  Switch1/1 -> Bus Creator/2  "DrvCmd"
  Bus Selector1/12 -> Bus Assignment1/13  "<DecelZero>"
  Bus Selector1/11 -> Bus Assignment1/12  "<DecelHld>"
  Bus Selector1/2 -> Unit Conversion1/1  "<SteerOvrCmd>"
  Bus Selector1/6 -> Bus Assignment1/7  "<AccelOvrCmd>"
  ExtDrvCmds/1 -> Bus Assignment1/1, Switch1/1
  ExtDrvRefSwitch/1 -> Switch/2
  ExtDrvCmdsSwitch/1 -> Switch1/2
  Switch/1 -> Bus Creator/1  "DrvRef"
  Bus Selector/4 -> Bus Assignment/7  "<CurvRef>"
  Bus Selector1/5 -> Bus Assignment1/6  "<EnblAccelOvr>"
  Bus Creator/1 -> VehRef/1  "VehRef"
  Unit Conversion1/1 -> Bus Assignment1/3
  Unit Conversion2/1 -> Bus Assignment/2

== system ConfiguredVirtualVehicleModel/Vehicle/Chassis Input ==
  Env : Inport
  Driver : Inport  Port=2
  Cntrl : Inport  Port=3
  Bus Selector1 : BusSelector  OutputSignals=Gnd.Z
  Bus Selector2 : BusSelector  OutputSignals=Wind
  Bus Selector3 : BusSelector  OutputSignals=Gnd.lambda_mux
  Bus Selector4 : BusSelector  OutputSignals=Grade
  Bus Selector5 : BusSelector  OutputSignals=SteerCmd
  Bus Selector6 : BusSelector  OutputSignals=Vcu.VcuBrkPrsCmd
  Bus Selector7 : BusSelector  OutputSignals=Gnd.DCM
  First Order Hold1 : FirstOrderHold  ErrorTolerance=inf
  Wind : Outport  VectorParamsAs1DForOutWhenUnconnected=off
  Gnd : Outport  Port=2  VectorParamsAs1DForOutWhenUnconnected=off
  Mu : Outport  Port=3  VectorParamsAs1DForOutWhenUnconnected=off
  Grade : Outport  Port=4  VectorParamsAs1DForOutWhenUnconnected=off
  GndDCM : Outport  Port=5  VectorParamsAs1DForOutWhenUnconnected=off
  SteerCmd : Outport  Port=6  VectorParamsAs1DForOutWhenUnconnected=off
  BrkPrsCmd : Outport  Port=7  VectorParamsAs1DForOutWhenUnconnected=off
  wires:
  Env/1 -> Bus Selector7/1, Bus Selector4/1, Bus Selector3/1, Bus Selector1/1, Bus Selector2/1
  Bus Selector2/1 -> Wind/1  "<Wind>"
  Driver/1 -> Bus Selector5/1
  Bus Selector5/1 -> SteerCmd/1  "<SteerCmd>"
  Cntrl/1 -> Bus Selector6/1
  Bus Selector6/1 -> First Order Hold1/1  "<VcuBrkPrsCmd>"
  Bus Selector4/1 -> Grade/1  "<Grade>"
  First Order Hold1/1 -> BrkPrsCmd/1
  Bus Selector7/1 -> GndDCM/1  "<DCM>"
  Bus Selector3/1 -> Mu/1  "<lambda_mux>"
  Bus Selector1/1 -> Gnd/1  "<Z>"

== system ConfiguredVirtualVehicleModel/Vehicle/Chassis Output ==
  Veh : Inport
  Wheels : Inport  Port=2
  Steering : Inport  Port=3
  Susp : Inport  Port=4
  Out Bus Element4 : Outport  PortName=VehFdbk
  Out Bus Element1 : Outport  Port=2  PortName=WheelsFdbk
  Out Bus Element2 : Outport  Port=3  PortName=SteeringFdbk
  Out Bus Element3 : Outport  Port=4  PortName=SuspensionFdbk
  wires:
  Veh/1 -> Out Bus Element4/1
  Wheels/1 -> Out Bus Element1/1
  Steering/1 -> Out Bus Element2/1
  Susp/1 -> Out Bus Element3/1

== system ConfiguredVirtualVehicleModel/Vehicle/Drivetrain Input ==
  Cntrl : Inport
  Bus Selector3 : BusSelector  OutputSignals=Trans.GearCmd,Vcu.Cltch1Cmd,Diff.DiffrntlPrsCmd
  First Order Hold1 : FirstOrderHold  ErrorTolerance=inf
  Rate Transition : RateTransition  InitialCondition=CtrlTcuInitGear
  Rate Transition1 : RateTransition  InitialCondition=CtrlVcuCltch1InitCmd
  GearCmd : Outport  VectorParamsAs1DForOutWhenUnconnected=off
  Cltch1Cmd : Outport  Port=2  VectorParamsAs1DForOutWhenUnconnected=off
  DiffrntlPrsCmd : Outport  Port=3  VectorParamsAs1DForOutWhenUnconnected=off
  wires:
  Cntrl/1 -> Bus Selector3/1
  Bus Selector3/1 -> Rate Transition/1  "<GearCmd>"
  Bus Selector3/3 -> First Order Hold1/1  "<DiffrntlPrsCmd>"
  Bus Selector3/2 -> Rate Transition1/1  "<Cltch1Cmd>"
  Rate Transition1/1 -> Cltch1Cmd/1
  First Order Hold1/1 -> DiffrntlPrsCmd/1
  Rate Transition/1 -> GearCmd/1

== system ConfiguredVirtualVehicleModel/Vehicle/Drivetrain Output ==
  AxlTrq : Inport
  EngSpd : Inport  Port=2
  DriveshftSpd : Inport  Port=3
  EMSpd : Inport  Port=4
  TransInfo : Inport  Port=5
  Bus Creator1 : BusCreator  Inputs=5
  Driveline : Outport  VectorParamsAs1DForOutWhenUnconnected=off
  wires:
  Bus Creator1/1 -> Driveline/1  "Driveline"
  DriveshftSpd/1 -> Bus Creator1/3  "DriveshftSpd"
  AxlTrq/1 -> Bus Creator1/1  "AxlTrq"
  EngSpd/1 -> Bus Creator1/2  "EngSpd"
  EMSpd/1 -> Bus Creator1/4  "EMSpd"
  TransInfo/1 -> Bus Creator1/5  "TransInfo"

== system ConfiguredVirtualVehicleModel/Vehicle/Electrical System Input ==
  Cntrl : Inport
  Env : Inport  Port=2
  Bus Selector : BusSelector  OutputSignals=AmbTemp
  Bus Selector2 : BusSelector  OutputSignals=Vcu.EMTrqCmd,Vcu.FuelCellCurrCmd,Vcu.FuelCellTempCmd,BMS
  First Order Hold : FirstOrderHold  ErrorTolerance=inf  AllowContinuousInput=on
  First Order Hold1 : FirstOrderHold  ErrorTolerance=inf  AllowContinuousInput=on
  First Order Hold2 : FirstOrderHold  ErrorTolerance=inf  AllowContinuousInput=on
  EMTrqCmd : Outport  VectorParamsAs1DForOutWhenUnconnected=off
  AmbTemp : Outport  Port=2  VectorParamsAs1DForOutWhenUnconnected=off
  FuelCellCurrCmd : Outport  Port=3  VectorParamsAs1DForOutWhenUnconnected=off
  FuelCellTempCmd : Outport  Port=4  VectorParamsAs1DForOutWhenUnconnected=off
  BMS : Outport  Port=5  VectorParamsAs1DForOutWhenUnconnected=off
  wires:
  Env/1 -> Bus Selector/1
  Bus Selector/1 -> AmbTemp/1  "<AmbTemp>"
  Cntrl/1 -> Bus Selector2/1
  Bus Selector2/1 -> First Order Hold/1  "<EMTrqCmd>"
  First Order Hold/1 -> EMTrqCmd/1  "EMTrqCmd"
  First Order Hold1/1 -> FuelCellCurrCmd/1  "FuelCellCurrCmd"
  First Order Hold2/1 -> FuelCellTempCmd/1  "FuelCellTempCmd"
  Bus Selector2/2 -> First Order Hold1/1  "<FuelCellCurrCmd>"
  Bus Selector2/3 -> First Order Hold2/1  "<FuelCellTempCmd>"
  Bus Selector2/4 -> BMS/1  "<BMS>"

== system ConfiguredVirtualVehicleModel/Vehicle/Electrical System Output ==
  Battery : Inport
  ElecMachine : Inport  Port=2
  FuelCell : Inport  Port=3
  Out Bus Element4 : Outport  PortName=BatteryFdbk
  Out Bus Element1 : Outport  Port=2  PortName=ElecMachineFdbk
  Out Bus Element2 : Outport  Port=3  PortName=FuelCellFdbk
  wires:
  Battery/1 -> Out Bus Element4/1
  ElecMachine/1 -> Out Bus Element1/1
  FuelCell/1 -> Out Bus Element2/1

== system ConfiguredVirtualVehicleModel/Vehicle/Engine Input ==
  Cntrl : Inport
  Bus Creator : BusCreator  Inputs=17
  Bus Selector : BusSelector  OutputSignals=Engine.ThrPosPctCmd,Engine.WgAreaPctCmd,Engine.InjPw,Engine.FuelMainSoi,Engine.SpkAdv,Engine.IntkCamPhaseCmd,Engine.ExhCamPhaseCmd,Engine.TurboRackPosCmd,Engine.EgrVlvAreaPctCmd,Engine.VarCompRatioPosCmd,Engine.IntkVlvLiftCmd,Engine.VarIntkRunLenCmd,Engine.ClsdLpFuelMult,Engine.IntkSwirlVlvPosCmd,Engine.TrqCmd,Engine.LoadCmd,Engine.EstIntkPortFlw
  First Order Hold{,1..16} (17 alike) : FirstOrderHold  ErrorTolerance=inf
  Engine : Outport
  wires:
  Bus Selector/14 -> First Order Hold14/1  "<IntkSwirlVlvPosCmd>"
  Bus Selector/12 -> First Order Hold13/1  "<VarIntkRunLenCmd>"
  Bus Selector/15 -> First Order Hold2/1  "<TrqCmd>"
  Bus Selector/13 -> First Order Hold/1  "<ClsdLpFuelMult>"
  Bus Selector/7 -> First Order Hold8/1  "<ExhCamPhaseCmd>"
  First Order Hold11/1 -> Bus Creator/10  "VarCompRatioPosCmd"
  Bus Selector/4 -> First Order Hold3/1  "<FuelMainSoi>"
  Bus Selector/8 -> First Order Hold9/1  "<TurboRackPosCmd>"
  Bus Selector/5 -> First Order Hold4/1  "<SpkAdv>"
  Bus Selector/9 -> First Order Hold10/1  "<EgrVlvAreaPctCmd>"
  Bus Selector/11 -> First Order Hold12/1  "<IntkVlvLiftCmd>"
  First Order Hold/1 -> Bus Creator/13  "ClsdLpFuelMult"
  Bus Selector/6 -> First Order Hold7/1  "<IntkCamPhaseCmd>"
  First Order Hold1/1 -> Bus Creator/3  "InjPw"
  First Order Hold7/1 -> Bus Creator/6  "IntkCamPhaseCmd"
  First Order Hold9/1 -> Bus Creator/8  "TurboRackPosCmd"
  Bus Selector/3 -> First Order Hold1/1  "<InjPw>"
  First Order Hold5/1 -> Bus Creator/1  "ThrPosPctCmd"
  First Order Hold3/1 -> Bus Creator/4  "FuelMainSoi"
  First Order Hold10/1 -> Bus Creator/9  "EgrVlvAreaPctCmd"
  First Order Hold12/1 -> Bus Creator/11  "IntkVlvLiftCmd"
  First Order Hold13/1 -> Bus Creator/12  "VarIntkRunLenCmd"
  First Order Hold2/1 -> Bus Creator/15  "TrqCmd"
  Bus Selector/1 -> First Order Hold5/1  "<ThrPosPctCmd>"
  Bus Selector/2 -> First Order Hold6/1  "<WgAreaPctCmd>"
  First Order Hold8/1 -> Bus Creator/7  "ExhCamPhaseCmd"
  First Order Hold6/1 -> Bus Creator/2  "WgAreaPctCmd"
  First Order Hold14/1 -> Bus Creator/14  "IntkSwirlVlvPosCmd"
  First Order Hold4/1 -> Bus Creator/5  "SpkAdv"
  Bus Selector/10 -> First Order Hold11/1  "<VarCompRatioPosCmd>"
  Bus Creator/1 -> Engine/1  "Engine"
  Cntrl/1 -> Bus Selector/1
  Bus Selector/16 -> First Order Hold15/1  "<LoadCmd>"
  Bus Selector/17 -> First Order Hold16/1  "<EstIntkPortFlw>"
  First Order Hold15/1 -> Bus Creator/16  "LoadCmd"
  First Order Hold16/1 -> Bus Creator/17  "EstIntkPortFlw"

== system ConfiguredVirtualVehicleModel/Vehicle/Engine Output ==
  "EngFdbk " : Inport
  EngFdbk : Outport  VectorParamsAs1DForOutWhenUnconnected=off
  wires:
  "EngFdbk "/1 -> EngFdbk/1  "EngFdbk"

== system ConfiguredVirtualVehicleModel/Vehicle/Pedal Cluster Input ==
  Driver : Inport
  Bus Selector : BusSelector  OutputSignals=SteerCmd,AccelCmd,DecelCmd,GearCmd,IgnSwtch,LightsCmd.HighBeamCmd,LightsCmd.LowBeamCmd,LightsCmd.LeftSignalCmd,LightsCmd.RightSignalCmd,LightsCmd.HazzardCmd
  SteerCmd : Outport  VectorParamsAs1DForOutWhenUnconnected=off
  AccelCmd : Outport  Port=2  VectorParamsAs1DForOutWhenUnconnected=off
  DecelCmd : Outport  Port=3  VectorParamsAs1DForOutWhenUnconnected=off
  DrvrGearCmd : Outport  Port=4  VectorParamsAs1DForOutWhenUnconnected=off
  IgnCmd : Outport  Port=5  VectorParamsAs1DForOutWhenUnconnected=off
  HighBeamCmd : Outport  Port=6  VectorParamsAs1DForOutWhenUnconnected=off
  LowBeamCmd : Outport  Port=7  VectorParamsAs1DForOutWhenUnconnected=off
  LeftSignalCmd : Outport  Port=8  VectorParamsAs1DForOutWhenUnconnected=off
  RightSignalCmd : Outport  Port=9  VectorParamsAs1DForOutWhenUnconnected=off
  HazzardCmd : Outport  Port=10  VectorParamsAs1DForOutWhenUnconnected=off
  wires:
  Bus Selector/2 -> AccelCmd/1  "<AccelCmd>"
  Driver/1 -> Bus Selector/1
  Bus Selector/3 -> DecelCmd/1  "<DecelCmd>"
  Bus Selector/4 -> DrvrGearCmd/1  "<GearCmd>"
  Bus Selector/1 -> SteerCmd/1  "<SteerCmd>"
  Bus Selector/5 -> IgnCmd/1  "<IgnSwtch>"
  Bus Selector/6 -> HighBeamCmd/1  "<HighBeamCmd>"
  Bus Selector/7 -> LowBeamCmd/1  "<LowBeamCmd>"
  Bus Selector/8 -> LeftSignalCmd/1  "<LeftSignalCmd>"
  Bus Selector/9 -> RightSignalCmd/1  "<RightSignalCmd>"
  Bus Selector/10 -> HazzardCmd/1  "<HazzardCmd>"

== system ConfiguredVirtualVehicleModel/Vehicle/Pedal Cluster Output ==
  Driver : Inport
  OperatorFdbk : Outport
  wires:
  Driver/1 -> OperatorFdbk/1

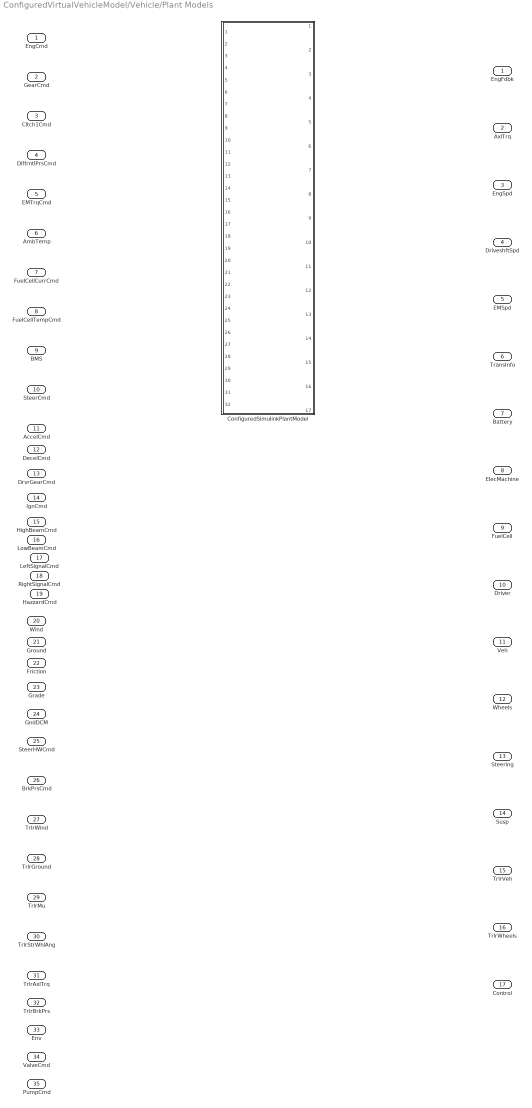
== system ConfiguredVirtualVehicleModel/Vehicle/Plant Models ==
  EngCmd : Inport
  GearCmd : Inport  Port=2
  Cltch1Cmd : Inport  Port=3
  DiffrntlPrsCmd : Inport  Port=4
  EMTrqCmd : Inport  Port=5
  AmbTemp : Inport  Port=6
  FuelCellCurrCmd : Inport  Port=7
  FuelCellTempCmd : Inport  Port=8
  BMS : Inport  Port=9
  SteerCmd : Inport  Port=10
  AccelCmd : Inport  Port=11
  DecelCmd : Inport  Port=12
  DrvrGearCmd : Inport  Port=13
  IgnCmd : Inport  Port=14
  HighBeamCmd : Inport  Port=15
  LowBeamCmd : Inport  Port=16
  LeftSignalCmd : Inport  Port=17
  RightSignalCmd : Inport  Port=18
  HazzardCmd : Inport  Port=19
  Wind : Inport  Port=20
  Ground : Inport  Port=21
  Friction : Inport  Port=22
  Grade : Inport  Port=23
  GndDCM : Inport  Port=24
  SteerHWCmd : Inport  Port=25
  BrkPrsCmd : Inport  Port=26
  TrlrWind : Inport  Port=27
  TrlrGround : Inport  Port=28
  TrlrMu : Inport  Port=29
  TrlrStrWhlAng : Inport  Port=30
  TrlrAxlTrq : Inport  Port=31
  TrlrBrkPrs : Inport  Port=32
  Env : Inport  Port=33
  ValveCmd : Inport  Port=34
  PumpCmd : Inport  Port=35
  ConfiguredSimulinkPlantModel : Subsystem  VariantControl=ConfiguredSimulinkPlantModel  ReferencedSubsystem=ConfiguredSimulinkPlantModel
  EngFdbk : Outport
  AxlTrq : Outport  Port=2
  EngSpd : Outport  Port=3
  DriveshftSpd : Outport  Port=4
  EMSpd : Outport  Port=5
  TransInfo : Outport  Port=6
  Battery : Outport  Port=7
  ElecMachine : Outport  Port=8
  FuelCell : Outport  Port=9
  Driver : Outport  Port=10
  Veh : Outport  Port=11
  Wheels : Outport  Port=12
  Steering : Outport  Port=13
  Susp : Outport  Port=14
  TrlrVeh : Outport  Port=15
  TrlrWheels : Outport  Port=16
  Control : Outport  Port=17

== system ConfiguredVirtualVehicleModel/Vehicle/Sensor Input ==
  EnvIn : Inport
  Env : Outport
  wires:
  EnvIn/1 -> Env/1  "Env"

== system ConfiguredVirtualVehicleModel/Vehicle/Sensor Output ==
  Control : Inport
  CntrlFdbk : Outport
  wires:
  Control/1 -> CntrlFdbk/1

== system ConfiguredVirtualVehicleModel/Vehicle/Thermal Input ==
  Cntrl : Inport
  Bus Selector : BusSelector  OutputSignals=Thermal.ValveCmd,Thermal.PumpCmd
  First Order Hold : FirstOrderHold  ErrorTolerance=inf
  First Order Hold1 : FirstOrderHold  ErrorTolerance=inf
  ValveCmd : Outport
  PumpCmd : Outport  Port=2
  wires:
  Bus Selector/2 -> First Order Hold1/1  "<PumpCmd>"
  Bus Selector/1 -> First Order Hold/1  "<ValveCmd>"
  First Order Hold/1 -> ValveCmd/1
  Cntrl/1 -> Bus Selector/1
  First Order Hold1/1 -> PumpCmd/1

== system ConfiguredVirtualVehicleModel/Vehicle/Trailer Input ==
  Env : Inport
  Cntrl : Inport  Port=2
  Bus Selector2 : BusSelector  OutputSignals=Wind
  Bus Selector4 : BusSelector  OutputSignals=Vcu.VcuTrlrBrkPrsCmd
  Constant1 : Constant  Value=zeros(2,1)
  Constant2 : Constant  Value=ones(2,1)
  Constant3 : Constant  Value=[0 0 0 0 0 0]
  Constant4 : Constant  Value=0
  Ground Info Trailer : Subsystem  Commented=on  Variant=on  VariantControlMode=label  VariantControl=Choice  LabelModeActiveChoice=0
  Terminator1 : Terminator
  Terminator2 : Terminator
  TrlrWind : Outport  VectorParamsAs1DForOutWhenUnconnected=off
  TrlrGnd : Outport  Port=2  VectorParamsAs1DForOutWhenUnconnected=off
  TrlrMu : Outport  Port=3  VectorParamsAs1DForOutWhenUnconnected=off
  TrlrStrWhlAng : Outport  Port=4  VectorParamsAs1DForOutWhenUnconnected=off
  TrlrAxlTrq : Outport  Port=5  VectorParamsAs1DForOutWhenUnconnected=off
  TrlrBrkPrs : Outport  Port=6  VectorParamsAs1DForOutWhenUnconnected=off
  wires:
  Bus Selector2/1 -> TrlrWind/1  "<Wind>"
  Env/1 -> Bus Selector2/1, Ground Info Trailer/1(Env)
  Constant3/1 -> TrlrStrWhlAng/1
  Constant4/1 -> TrlrAxlTrq/1
  Bus Selector4/1 -> TrlrBrkPrs/1  "<VcuTrlrBrkPrsCmd>"
  Cntrl/1 -> Bus Selector4/1
  Constant2/1 -> TrlrMu/1
  Constant1/1 -> TrlrGnd/1
  Ground Info Trailer/1(Ground) -> Terminator1/1
  Ground Info Trailer/2(Friction) -> Terminator2/1

== system ConfiguredVirtualVehicleModel/Vehicle/Trailer Output ==
  Veh : Inport
  Wheels : Inport  Port=2
  Out Bus Element4 : Outport  PortName=VehFdbk
  Out Bus Element1 : Outport  Port=2  PortName=WheelsFdbk
  wires:
  Wheels/1 -> Out Bus Element1/1
  Veh/1 -> Out Bus Element4/1

== system ConfiguredVirtualVehicleModel/Visualization/Coordinate Systems ==
  VehFdbkIn : Inport
  ISO 8855 (Z-up) : Subsystem  VariantControl=Choice
  SAE J670 (Z-down) : Subsystem  VariantControl=ISO 8855 (Z-up)1
  VehFdbk : Outport

== system ConfiguredVirtualVehicleModel/Visualization/DataLogging ==
  VehFdbk : Inport
  Bus Selector : BusSelector  OutputSignals=Battery.BattSoc,Battery.BattVolt,Battery.BattCurr,Body.BdyFrm.Cg.Vel.xdot,Body.BdyFrm.Cg.Acc.ax,Body.BdyFrm.Cg.Acc.ay,Body.BdyFrm.Cg.Acc.az,Driver.SteerFdbk,Driver.AccelFdbk,Driver.DecelFdbk,Driver.GearFdbk,Driveline.EMSpd,EM.EMTrq
  Terminator{,1..12} (13 alike) : Terminator
  wires:
  VehFdbk/1 -> Bus Selector/1
  Bus Selector/10 -> Terminator9/1  "<DecelFdbk>"
  Bus Selector/1 -> Terminator/1  "<BattSoc>"
  Bus Selector/2 -> Terminator1/1  "<BattVolt>"
  Bus Selector/3 -> Terminator2/1  "<BattCurr>"
  Bus Selector/4 -> Terminator3/1  "<xdot>"
  Bus Selector/5 -> Terminator4/1  "<ax>"
  Bus Selector/13 -> Terminator12/1  "<EMTrq>"
  Bus Selector/11 -> Terminator10/1  "<GearFdbk>"
  Bus Selector/6 -> Terminator5/1  "<ay>"
  Bus Selector/8 -> Terminator7/1  "<SteerFdbk>"
  Bus Selector/7 -> Terminator6/1  "<az>"
  Bus Selector/9 -> Terminator8/1  "<AccelFdbk>"
  Bus Selector/12 -> Terminator11/1  "<EMSpd>"
